simulink model "two_states_with_trigger_and_complex_condition"  (R2017b)
settings: Solver=FixedStepDiscrete  StartTime=0.0  StopTime=10.0  RelTol=1e-3
settings Model: Creator=flosch  LastModifiedBy=flosch
settings ConfigComp: CovScope=ReferencedModels  CovIncludeTopModel=off

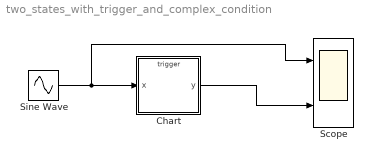
== system two_states_with_trigger_and_complex_condition ==
  Chart : Stateflow chart  TreatAsAtomicUnit=on
  Scope : Scope  NumInputPorts=2
  Sine Wave : Sin  SampleTime=0
  wires:
  Sine Wave/1 -> Scope/1, Chart/1(x)
  Chart/1(y) -> Scope/2

== stateflow chart two_states_with_trigger_and_complex_condition/Chart ==
  state Potato
    entry: y = x;
  state Kitten
    entry: y = 0;
  note: cyc = 5
      | obj = 4
      | lines = 4
  (default) -> Potato
  Potato -> Kitten : Event_A[x > 2 && x < 5]
  data: t0 constant double =0.0; x input; y output
  events: Event_A input FUNCTION_CALL_EVENT
